simulink model "SensingSubsystem"  (R2026a)
settings: Solver=ode15s  StopTime=10  FixedStep=1e-3  MaxStep=1e-6  RelTol=1e-5
model workspace (MAT data in the model file):
  SL_ROS_VariableLengthArrays_MaxSizes : object (value not decoded)
undefined symbols (not defined in the file or in its folder): AS7341_8Channel, BPW34_Photodiode, DS18B20_Temperature, MS5837_Pressure, sandy_sensors
libraries: fl_lib x32, nesl_utility x22, ee_lib x6, ros2lib x4
(part 2 of 2)

== matlab function SensingSubsystem/AS7341_8Channel/RGB_to_F1F8 ==
  data: msg input Bus: SL_Bus_sensor_msgs_Image; F output
function F = rgb_to_bands(msg)
%#codegen
% Synthesise 8 AS7341 channels (F1..F8) from a Gazebo RGB image.
% Output F is uint16 1x8, range 0..65535, matching AS7341 ADC.

F = uint16(zeros(1, 8));
n = numel(msg.data);

if mod(n, 3) == 0 && n > 0
    d = double(msg.data);
    R = mean(d(1:3:end));
    G = mean(d(2:3:end));
    B = mean(d(3:3:end));

    % 8x3 weight matrix (rows = F1..F8, cols = R G B)
    W = [0.00 0.05 0.95;   % F1 415nm
        0.00 0.10 0.90;   % F2 445nm
        0.00 0.25 0.75;   % F3 480nm
        0.00 0.50 0.50;   % F4 515nm
        0.10 0.80 0.10;   % F5 555nm
        0.30 0.65 0.05;   % F6 590nm
        0.75 0.25 0.00;   % F7 630nm
        0.95 0.05 0.00];  % F8 680nm

    bands = W * [R; G; B];
    F = uint16(min(65535, bands * 257));
end
end
